simulink model "ex6sim"  (R2015a)
settings: Solver=ode45  StartTime=0.0  StopTime=10.0  RelTol=1e-3
settings Model: Creator=brunopeixoto  LastModifiedBy=brunopeixoto

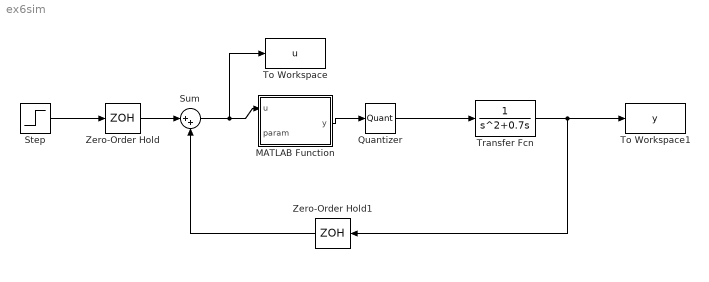
== system ex6sim ==
  MATLAB Function : MATLAB Function  TreatAsAtomicUnit=on
  Quantizer : Quantizer
  Step : Step  SampleTime=0
  Sum : Sum  Inputs=|++
  To Workspace : ToWorkspace  VariableName=u  SaveFormat=Structure With Time  SampleTime=-1
  To Workspace1 : ToWorkspace  VariableName=y  SaveFormat=Structure With Time  SampleTime=-1
  Transfer Fcn : TransferFcn  Denominator=[1 0.7 0]
  Zero-Order Hold : ZeroOrderHold
  Zero-Order Hold1 : ZeroOrderHold
  wires:
  Step/1 -> Zero-Order Hold/1
  Zero-Order Hold/1 -> Sum/1
  Transfer Fcn/1 -> To Workspace1/1, Zero-Order Hold1/1
  MATLAB Function/1(y) -> Quantizer/1
  Sum/1 -> To Workspace/1, MATLAB Function/1(u)
  Quantizer/1 -> Transfer Fcn/1
  Zero-Order Hold1/1 -> Sum/2

== matlab function ex6sim/MATLAB Function ==
  data: u input; y output; param input
function y = fcn(u, param)
%#codegen

Cz = param(1);

y = u;
